simulink model "lab3"  (R2018b)
settings: Solver=ode23tb  StartTime=0.0  StopTime=4.0  MaxStep=5e-006  RelTol=1e-3
libraries: powerlib x6, powerlib_extras x2, simulink x1
settings Model: Creator=KJ_Fa  LastModifiedBy=yangr
settings SolverCC: MaxConsecutiveZCs=1000000  ZeroCrossAlgorithm=Adaptive
settings DebuggingCC: LibraryContextMissingDiagnostic=none
settings SFSimCC: SimUseLocalCustomCode=off
settings RTWCC: RTWUseLocalCustomCode=off
settings CodeAppCC: StateflowObjectComments=on

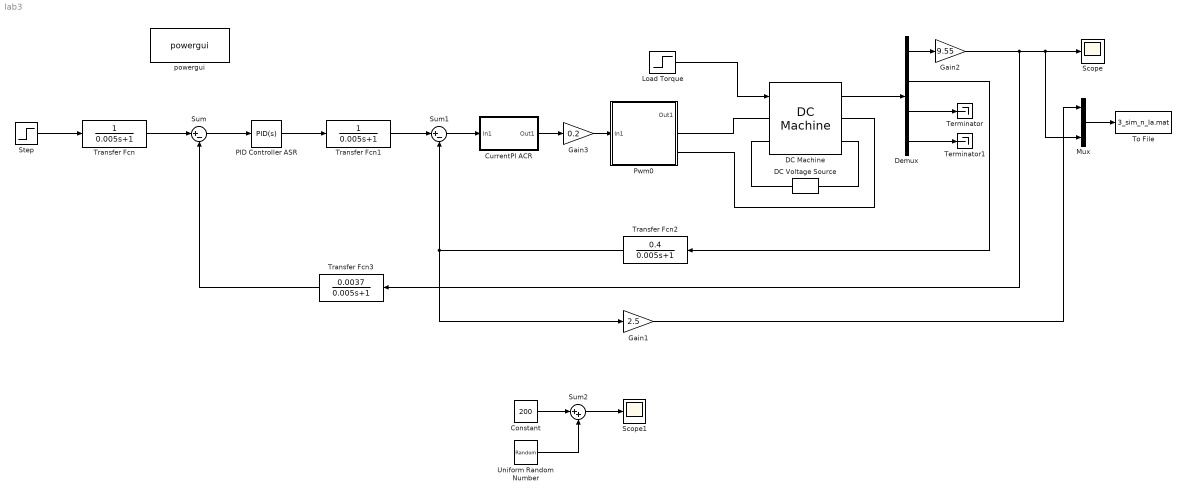
== system lab3 ==
  Constant : Constant  Value=200
  CurrentPI ACR : Subsystem
  DC Machine : powerlib/Machines/DC Machine  PresetModel=No  MechanicalLoad=Torque TL  FieldType=Wound  ShowDetailedParameters=on  MeasurementBus=off  RLa="[ 1.92  0.01]"  RLf="[ 220  120]"  Laf=1.25  MachineConstant=Torque constant (N.m/A)  Ke=1.8  Kt=1.8  J=0.204  Bm=0.01  Tf=2  w0=0.1  Ifinit=1  TsPowergui=0  TsBlock=-1
      settings: SourceProductName=Simscape Electrical
  DC Voltage Source : powerlib/Electrical Sources/DC Voltage Source  Amplitude=200  Measurements=None
      settings: SourceProductName=Simscape Electrical
  Demux : Demux
  Gain1 : Gain  Gain=2.5
  Gain2 : Gain  Gain=9.55
  Gain3 : Gain  Gain=0.2
  Load Torque : Step  Time=3  Before=6  After=12  SampleTime=0
  Mux : Mux  Inputs=3
  PID Controller ASR : simulink/Continuous/PID Controller  Controller=PID  Form=Parallel  TimeDomain=Continuous-time  SampleTime=-1  IntegratorMethod=Forward Euler  FilterMethod=Forward Euler  ControllerParametersSource=internal  P=80.98  I=1079.73  D=0  UseFilter=on  N=100  TunerSelectOption=Transfer Function Based (PID Tuner App)  InitialConditionSource=internal  InitialConditionForIntegrator=0  InitialConditionForFilter=0  DifferentiatorICPrevScaledInput=0  ExternalReset=none  TrackingMode=off  Kt=1  LimitOutput=on  UpperSaturationLimit=8  LowerSaturationLimit=-8  LinearizeAsGain=on  AntiWindupMode=clamping  Kb=1  POutMin=[]  POutMax=[]  IOutMin=[]  IOutMax=[]  DOutMin=[]  DOutMax=[]  NOutMin=[]  NOutMax=[]  SumOutMin=[]  SumOutMax=[]  SaturationOutMin=[]  SaturationOutMax=[]  PParamMin=[]  PParamMax=[]  IParamMin=[]  IParamMax=[]  DParamMin=[]  DParamMax=[]  NParamMin=[]  NParamMax=[]  KbParamMin=[]  KbParamMax=[]  KtParamMin=[]  KtParamMax=[]  KbOutMin=[]  KbOutMax=[]  KtOutMin=[]  KtOutMax=[]  IntegratorOutMin=[]  IntegratorOutMax=[]  FilterOutMin=[]  FilterOutMax=[]  SumI1OutMin=[]  SumI1OutMax=[]  SumI2OutMin=[]  SumI2OutMax=[]  SumI3OutMin=[]  SumI3OutMax=[]  SumI4OutMin=[]  SumI4OutMax=[]  SumDOutMin=[]  SumDOutMax=[]  DifferentiatorOutMin=[]  DifferentiatorOutMax=[]  FilterDiffOutCoefMin=[]  FilterDiffOutCoefMax=[]  ReciprocalOutMin=[]  ReciprocalOutMax=[]  SumDenOutMin=[]  SumDenOutMax=[]  SumNumOutMin=[]  SumNumOutMax=[]  DivideOutMin=[]  DivideOutMax=[]  IntegratorContinuousStateAttributes=''  IntegratorStateMustResolveToSignalObject=off  IntegratorRTWStateStorageClass=Auto  FilterContinuousStateAttributes=''  FilterStateMustResolveToSignalObject=off  FilterRTWStateStorageClass=Auto  ParallelPVariant=InternalParameters  IdealPVariant=Disabled  IVariant=InternalParameters  DVariant=InternalParameters  IntegratorVariant=Continuous  SatVariant=Enabled  AWVariant=ContClampingParallel  PCopyVariant=Disabled  TRVariant=Disabled  FdbkBlocksVariant=Forward  IdealPFdbkVariant=Disabled  SatFdbkVariant=Disabled  DerivativeFilterVariant=ContFilter  NVariant=InternalParameters  NCopyVariant=Disabled  FilterICVariant=InternalICsFilter  IntegratorICVariant=InternalICs  ExternalResetVariant=Disabled  TRSumVariant=Passthrough  SumFdbkVariant=Disabled  SumVariant=Sum_PID
  Pwm0 : Subsystem
  Scope : Scope
  Scope1 : Scope
  Step : Step  Time=0  After=5  SampleTime=0
  Sum : Sum  Inputs=|+-
  Sum1 : Sum  Inputs=|+-
  Sum2 : Sum  Inputs=|++
  Terminator : Terminator
  Terminator1 : Terminator
  To File : ToFile  Filename=3_sim_n_Ia.mat  MatrixName=signals
  Transfer Fcn : TransferFcn  Denominator=[0.005 1]
  Transfer Fcn1 : TransferFcn  Denominator=[0.005 1]
  Transfer Fcn2 : TransferFcn  Numerator=[0.4]  Denominator=[0.005 1]
  Transfer Fcn3 : TransferFcn  Numerator=[0.0037]  Denominator=[0.005 1]
  Uniform Random Number : UniformRandomNumber  Minimum=-50  Maximum=50  SampleTime=0.1
  powergui : powerlib/powergui  Priority=1  SimulationMode=Continuous  SampleTime=50e-6  frequency=60  Iterations=50  frequencyindice=0  Pbase=100e6  ErrMax=1e-4  UnitsV=kV  UnitsW=MW  buscounter=0  FunctionMessages=off  echomessages=off  EnableUseOfTLC=off  CurrentSourceSwitches=off  DisableSnubberDevices=off  DisableRonSwitches=off  DisableVfSwitches=off  DisplayEquations=off  SolverType=Tustin/Backward Euler (TBE)  Interpol=off  ExternalGateDelay=off  methode=off  Ts=100  x0status=blocks  SPID=on  SwTol=0  HookPort=off  RestoreLinks=warning  ResistiveCurrentMeasurement=off  Frange=[0:2:500]  Ylog=off  Xlog=on  ShowGrid=off  save=off  variable=ZData  structure=0  ZoomFFT=off  StartTime=0.0  cycles=1  DisplayStyle=1  fundamental=60  FreqAxis=off  MaxFrequency=1000  frequencyindicesteady=1  RmsSteady=1  display=off
  wires:
  Load Torque/1 -> DC Machine/1
  Demux/3 -> Terminator/1
  Demux/4 -> Terminator1/1
  Transfer Fcn2/1 -> Sum1/2, Gain1/1
  Demux/2 -> Transfer Fcn2/1
  Demux/1 -> Gain2/1
  DC Machine/1 -> Demux/1
  Gain2/1 -> Mux/3, Scope/1, Transfer Fcn3/1
  Transfer Fcn3/1 -> Sum/2
  Step/1 -> Transfer Fcn/1
  Transfer Fcn/1 -> Sum/1
  Sum/1 -> PID Controller ASR/1
  PID Controller ASR/1 -> Transfer Fcn1/1
  Transfer Fcn1/1 -> Sum1/1
  Sum1/1 -> CurrentPI ACR/1(In1)
  CurrentPI ACR/1(Out1) -> Gain3/1
  Mux/1 -> To File/1
  Gain3/1 -> Pwm0/1(In1)
  Gain1/1 -> Mux/1
  Constant/1 -> Sum2/1
  Uniform Random Number/1 -> Sum2/2
  Sum2/1 -> Scope1/1
  connections:
  Pwm0/RConn1 -- DC Machine/LConn1
  DC Machine/RConn1 -- Pwm0/RConn2
  DC Machine/LConn2 -- DC Voltage Source/RConn1
  DC Machine/RConn2 -- DC Voltage Source/LConn1

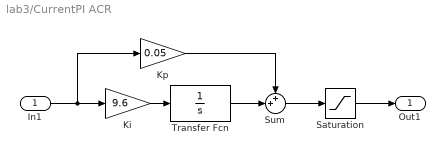
== system lab3/CurrentPI ACR ==
  In1 : Inport
  "Ki " : Gain  Gain=9.6
  Kp : Gain  Gain=0.05
  Saturation : Saturate  UpperLimit=5  LowerLimit=-5
  Sum : Sum  Inputs=++|
  Transfer Fcn : TransferFcn  Denominator=[1 0]
  Out1 : Outport
  wires:
  In1/1 -> Kp/1, "Ki "/1
  "Ki "/1 -> Transfer Fcn/1
  Kp/1 -> Sum/1
  Transfer Fcn/1 -> Sum/2
  Sum/1 -> Saturation/1
  Saturation/1 -> Out1/1

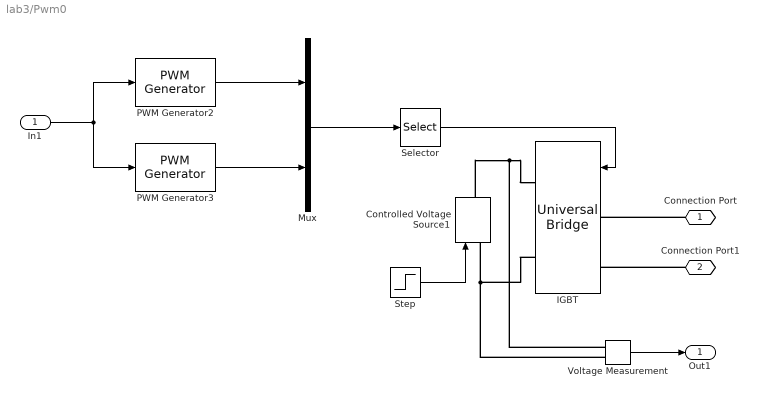
== system lab3/Pwm0 ==
  In1 : Inport
  Controlled Voltage Source1 : powerlib/Electrical Sources/Controlled Voltage Source  Initialize=on  Source_Type=DC  Amplitude=0  Phase=0  Frequency=0  Measurements=None
      settings: SourceProductName=Simscape Electrical
  IGBT : powerlib/Power Electronics/Universal Bridge  Arms=2  SnubberResistance=1e5  SnubberCapacitance=inf  Device=IGBT / Diodes  Ron=1e-3  Lon=0  ForwardVoltages="[  0  0  ]"  ForwardVoltage=0  GTOparameters=[ 10e-6 , 20e-6 ]  IGBTparameters=[ 1e-6 , 2e-6 ]  Measurements=None  Measurements_2=None  converterType=Rectifier
      settings: SourceProductName=Simscape Electrical
  Mux : Mux  Inputs=2
  PWM Generator2 : powerlib_extras/Control  Blocks/PWM Generator  GeneratorMode="1-arm  bridge (2 pulses)"  Fc=10800  Internal=off  mIndex=0.4  Freq=60  Phase=0
  PWM Generator3 : powerlib_extras/Control  Blocks/PWM Generator  GeneratorMode="1-arm  bridge (2 pulses)"  Fc=10800  Internal=off  mIndex=0.4  Freq=60  Phase=0
  Selector : Selector  InputPortWidth=4  IndexOptions=Index vector (dialog)  Indices=[1 2 4 3]  OutputSizes=1
  Step : Step  Time=0  After=250  SampleTime=0
  Voltage Measurement : powerlib/Measurements/Voltage Measurement  PhasorSimulation=off  OutputType=Complex  PSBequivalent=0
      settings: SourceProductName=Simscape Electrical
  Connection Port : PMIOPort  Side=Right
  Connection Port1 : PMIOPort  Port=2  Side=Right
  Out1 : Outport
  wires:
  Mux/1 -> Selector/1
  Selector/1 -> IGBT/1
  In1/1 -> PWM Generator2/1, PWM Generator3/1
  PWM Generator2/1 -> Mux/1
  PWM Generator3/1 -> Mux/2
  Step/1 -> Controlled Voltage Source1/1
  Voltage Measurement/1 -> Out1/1
  connections:
  Controlled Voltage Source1/RConn1 -- Voltage Measurement/LConn1 -- IGBT/RConn1
  IGBT/RConn2 -- Voltage Measurement/LConn2 -- Controlled Voltage Source1/LConn1
  Connection Port1/RConn1 -- IGBT/LConn2
  Connection Port/RConn1 -- IGBT/LConn1
